simulink model "lab6_non_lin"  (R2019b)
settings: Solver=VariableStepAuto  StartTime=0.0  StopTime=10.0  RelTol=1e-3
settings Model: Creator=Michał  LastModifiedBy=Michał

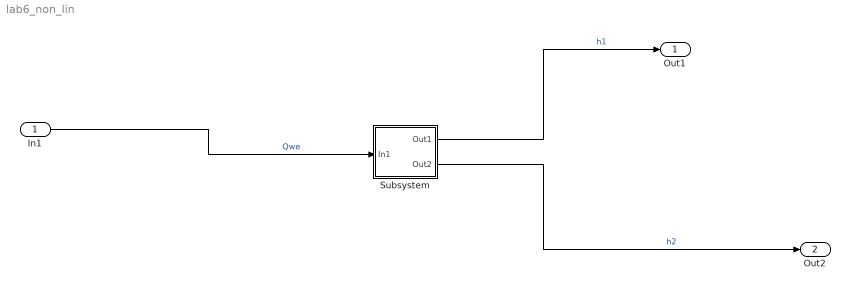
== system lab6_non_lin ==
  In1 : Inport
  Subsystem : Subsystem  mask{S1=0, S2=0, Swy1=0, Swy2=0, phi1=0, phi2=0, g=0, h1=0, h2=0}
  Out1 : Outport
  Out2 : Outport  Port=2
  wires:
  In1/1 -> Subsystem/1(In1)  "Qwe"
  Subsystem/1(Out1) -> Out1/1  "h1"
  Subsystem/2(Out2) -> Out2/1  "h2"

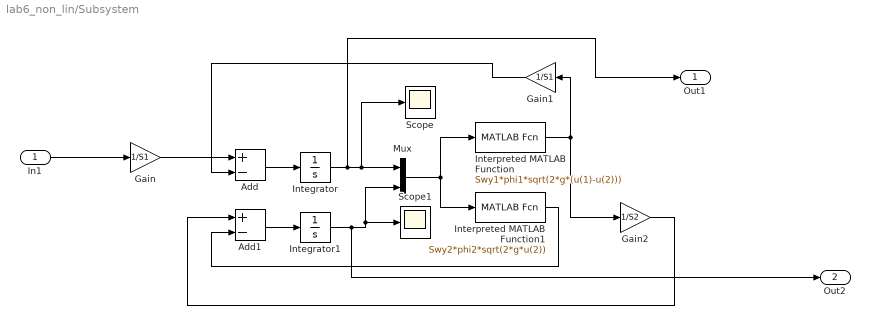
== system lab6_non_lin/Subsystem ==
  In1 : Inport
  Add : Sum  Inputs=+-
  Add1 : Sum  Inputs=+-
  Gain : Gain  Gain=1/S1
  Gain1 : Gain  Gain=1/S1
  Gain2 : Gain  Gain=1/S2
  Integrator : Integrator  InitialCondition=h1
  Integrator1 : Integrator  InitialCondition=h2
  Interpreted MATLAB Function : MATLABFcn  MATLABFcn=Swy1*phi1*sqrt(2*g*(u(1)-u(2)))
  Interpreted MATLAB Function1 : MATLABFcn  MATLABFcn=Swy2*phi2*sqrt(2*g*u(2))
  Mux : Mux  Inputs=2
  Scope : Scope
  Scope1 : Scope
  Out1 : Outport
  Out2 : Outport  Port=2
  wires:
  Add1/1 -> Integrator1/1
  Gain2/1 -> Add1/1
  Interpreted MATLAB Function/1 -> Gain1/1, Gain2/1
  In1/1 -> Gain/1
  Interpreted MATLAB Function1/1 -> Add1/2
  Integrator1/1 -> Out2/1, Scope1/1, Mux/2
  Integrator/1 -> Out1/1, Scope/1, Mux/1
  Mux/1 -> Interpreted MATLAB Function1/1, Interpreted MATLAB Function/1
  Gain1/1 -> Add/2
  Add/1 -> Integrator/1
  Gain/1 -> Add/1
